simulink model "lab65"  (R2023b)
settings: Solver=VariableStepAuto  StartTime=0.0  StopTime=20  RelTol=1e-3
undefined symbols (not defined in the file or in its folder): ki_FIM, kp_FIM
settings Model: Creator=Настя  LastModifiedBy=killer
settings SolverCC: AlgebraicLoopSolver=TrustRegion
settings DebuggingCC: UnconnectedInputMsg=warning  UnconnectedOutputMsg=warning  UnconnectedLineMsg=warning
settings ModelReferenceCC: EnableRefExpFcnMdlSchedulingChecks=on
settings RTWCC: DLArmComputeVersion=19.05

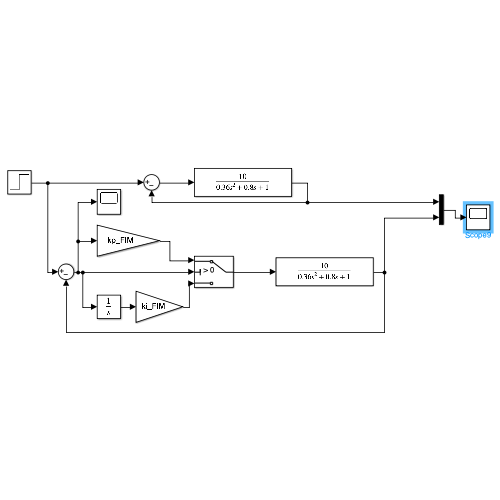
[thumbnail: Simulink's stored preview of the top-level diagram]
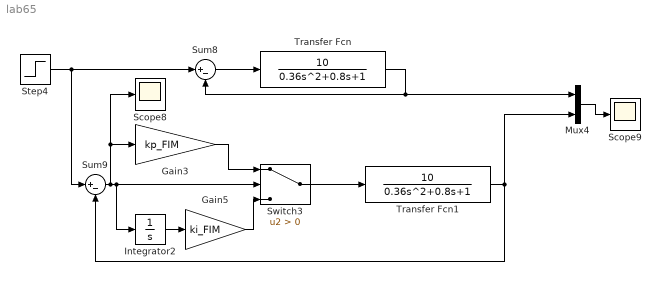
== system lab65 ==
  Gain3 : Gain  Gain=kp_FIM
  Gain5 : Gain  Gain=ki_FIM
  Integrator2 : Integrator
  Mux4 : Mux  Inputs=2
  Scope8 : Scope
  Scope9 : Scope
  Step4 : Step  Time=0  SampleTime=0
  Sum8 : Sum  Inputs=|+-
  Sum9 : Sum  Inputs=|+-
  Switch3 : Switch  Criteria=u2 > Threshold  SaturateOnIntegerOverflow=off  InputSameDT=off
  Transfer Fcn : TransferFcn  Numerator=[10]  Denominator=[0.36 0.8 1]
  Transfer Fcn1 : TransferFcn  Numerator=[10]  Denominator=[0.36 0.8 1]
  wires:
  Transfer Fcn/1 -> Sum8/2, Mux4/1
  Sum8/1 -> Transfer Fcn/1
  Integrator2/1 -> Gain5/1
  Step4/1 -> Sum8/1, Sum9/1
  Switch3/1 -> Transfer Fcn1/1
  Gain5/1 -> Switch3/3
  Mux4/1 -> Scope9/1
  Transfer Fcn1/1 -> Sum9/2, Mux4/2
  Sum9/1 -> Scope8/1, Gain3/1, Switch3/2, Integrator2/1
  Gain3/1 -> Switch3/1
